simulink model "Z_1Dctrl"  (R2023a)
settings: Solver=ode1  StartTime=0.0  StopTime=inf  FixedStep=0.001  RelTol=1e-3  EnableMultiTasking=on
PostLoadFcn:
  | , if any(exist('dsrtsu_mdlpostloadfcn', 'file') ~= 0), dsrtsu_mdlpostloadfcn('Execute', bdroot); end,
InitFcn:
  | , if any(exist('rtifpga_mdlclblib', 'file') ~= 0), rtifpga_mdlclblib('Init', bdroot); end,
  | [b,a] = butter(6,0.6)
  | z0_default = 0.080001
  | fatness_default = 1
  | offset_default = 0
  | scale_default = 0
  | tic
model workspace (MAT data in the model file):
  Iters = 5
  N_coils = 6
  fatness_default = 1
  running = 0
  z0_default = 0.080001
undefined symbols (not defined in the file): a, b, DiscIntNeverNeededParam
libraries: dspstat3 x11, simulink x5, commfilt2 x4, rti2004lib x3, rtilibm x1
(part 2 of 2)

== system Z_1Dctrl/get_plant_input/detect_stability/speed_and_position_testing_xy ==
  x : Inport
  y : Inport  Port=2
  speed analysis : Subsystem
  |vxy| comfort threshold : Constant  Value=1e-6
  x_converged : Outport
  y_converged : Outport  Port=2
  wires:
  x/1 -> speed analysis/1(x)
  |vxy| comfort threshold/1 -> speed analysis/3(vxy comfort threshold)
  speed analysis/2(vy low enough) -> y_converged/1
  speed analysis/1(vx low enough) -> x_converged/1
  y/1 -> speed analysis/2(y)

== system Z_1Dctrl/plant/Position Determination1/XY position Calculation ==
  note: !!MODIFIED!!
      | Before: "X_p, Y_p = Head2_read, Head3_read - radius_m".
      | After: "Head2_p, Head3_p = Head2_read, Head3_read + radius_m".
  note: Laser sensors output a voltage in [-10,10]V, proportional to the detected object's position in their 40mm FOV.
      | Conventions:
      | - Top of sensor (with large chamfer) is "up". Bottom of sensor is "down".
      | - "Upmost" measurement is -10V (-0.02m).
      | - "Downmost" measurement is +10V (+0.02m).
      | - Measurements go wonky if outer boundaries (+10V, -10V) are reached. For safety, do not let the magnet reach this range.
  Head II (Voltage) : Inport
  Head III (Voltage) : Inport  Port=2
  diameter_m : Inport  Port=3
  Mux : Mux  Inputs=2
  Sum : Sum  Inputs=|++
  Sum1 : Sum  Inputs=++|
  X_m : Fcn  Expr=(u(1)+u(2))*sin(pi/4)
  Y_m : Fcn  Expr=(u(1)-u(2))*sin(pi/4)
  diameter_to_radius : Gain  Gain=1/2
  volt_to_m : Gain  Gain=2/1000
  volt_to_m_2 : Gain  Gain=2/1000
  X_Position(m) : Outport
  Y_Position(m) : Outport  Port=2
  wires:
  Head III (Voltage)/1 -> volt_to_m_2/1
  Y_m/1 -> Y_Position(m)/1
  X_m/1 -> X_Position(m)/1
  Head II (Voltage)/1 -> volt_to_m/1
  Mux/1 -> Y_m/1, X_m/1
  Sum1/1 -> Mux/2  "Head3_p"
  volt_to_m_2/1 -> Sum1/2
  Sum/1 -> Mux/1  "Head2_p"
  diameter_to_radius/1 -> Sum1/1, Sum/2  "radius_m"
  volt_to_m/1 -> Sum/1
  diameter_m/1 -> diameter_to_radius/1

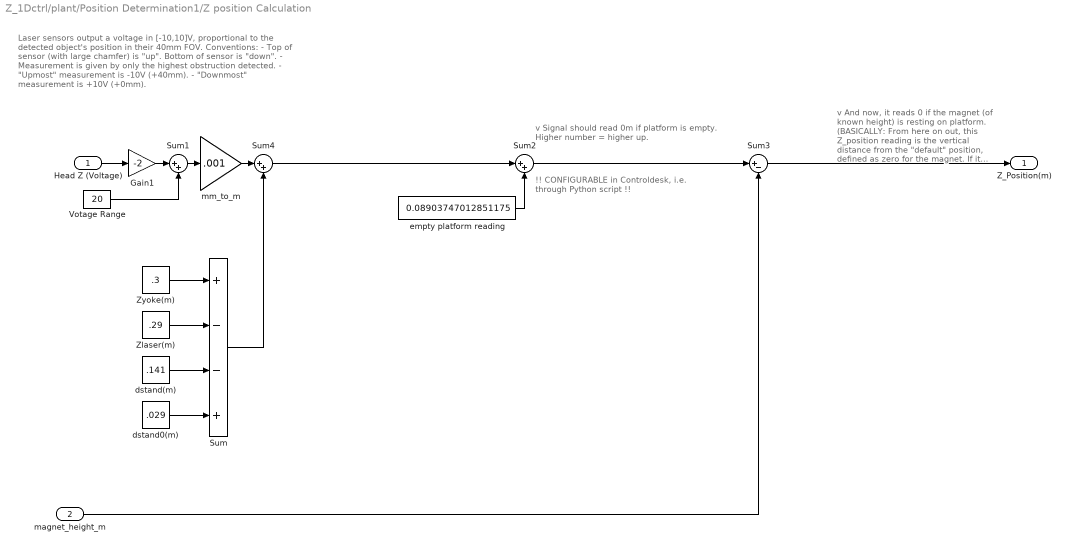
== system Z_1Dctrl/plant/Position Determination1/Z position Calculation ==
  note: Laser sensors output a voltage in [-10,10]V, proportional to the detected object's position in their 40mm FOV.
      | Conventions:
      | - Top of sensor (with large chamfer) is "up". Bottom of sensor is "down".
      | - Measurement is given by only the highest obstruction detected.
      | - "Upmost" measurement is -10V (+40mm).
      | - "Downmost" measurement is +10V (+0mm).
  note: v Signal should read 0m if platform is empty.
      | Higher number = higher up.
  note: v And now, it reads 0 if the magnet (of known height) is resting on platform.
      |
      | (BASICALLY: From here on out, this Z_position reading is the vertical distance from the "default" position, defined as zero for the magnet. If it reads something significantly different from 0, then double check the magnet height.)
  note: !! CONFIGURABLE in Controldesk, i.e. through Python script !!
  Head Z (Voltage) : Inport
  magnet_height_m : Inport  Port=2
  Gain1 : Gain  Gain=-2
  Sum : Sum  Inputs=+--+
  Sum1 : Sum  Inputs=|++
  Sum2 : Sum  Inputs=|++
  Sum3 : Sum  Inputs=|+-
  Sum4 : Sum  Inputs=|++
  Votage Range : Constant  Value=20
  Zlaser(m) : Constant  Value=.29
  Zyoke(m) : Constant  Value=.3
  dstand(m) : Constant  Value=.141
  dstand0(m) : Constant  Value=.029
  empty platform reading : Constant  Value=0.08903747012851175
  mm_to_m : Gain  Gain=.001
  Z_Position(m) : Outport
  wires:
  Sum2/1 -> Sum3/1
  Head Z (Voltage)/1 -> Gain1/1
  Sum/1 -> Sum4/2
  Sum1/1 -> mm_to_m/1
  Votage Range/1 -> Sum1/2
  Gain1/1 -> Sum1/1
  Zlaser(m)/1 -> Sum/2
  Zyoke(m)/1 -> Sum/1
  dstand(m)/1 -> Sum/3
  dstand0(m)/1 -> Sum/4
  magnet_height_m/1 -> Sum3/2
  Sum4/1 -> Sum2/1
  mm_to_m/1 -> Sum4/1
  empty platform reading/1 -> Sum2/2
  Sum3/1 -> Z_Position(m)/1

== system Z_1Dctrl/plant/Position Determination1/x filter ==
  u_raw : Inport
  10ms mean : Subsystem
  butter : DiscreteTransferFcn  Numerator=b  Denominator=a
  enable_butterworth : Constant
  enable_moving_mean : Constant
  switch_butter : Switch  Criteria=u2 > Threshold  SaturateOnIntegerOverflow=off  InputSameDT=off
  switch_movingmean : Switch  Criteria=u2 > Threshold  SaturateOnIntegerOverflow=off  InputSameDT=off
  u_filtered : Outport
  wires:
  enable_butterworth/1 -> switch_butter/2
  butter/1 -> switch_butter/1
  u_raw/1 -> switch_butter/3, butter/1
  enable_moving_mean/1 -> switch_movingmean/2
  switch_butter/1 -> 10ms mean/1(u), switch_movingmean/3
  10ms mean/1(movingmean(u)) -> switch_movingmean/1
  switch_movingmean/1 -> u_filtered/1

== system Z_1Dctrl/plant/Position Determination1/y filter ==
  u_raw : Inport
  10ms mean : Subsystem
  butter : DiscreteTransferFcn  Numerator=b  Denominator=a
  enable_butterworth : Constant
  enable_moving_mean : Constant
  switch_butter : Switch  Criteria=u2 > Threshold  SaturateOnIntegerOverflow=off  InputSameDT=off
  switch_movingmean : Switch  Criteria=u2 > Threshold  SaturateOnIntegerOverflow=off  InputSameDT=off
  u_filtered : Outport
  wires:
  enable_butterworth/1 -> switch_butter/2
  butter/1 -> switch_butter/1
  u_raw/1 -> switch_butter/3, butter/1
  enable_moving_mean/1 -> switch_movingmean/2
  switch_butter/1 -> 10ms mean/1(u), switch_movingmean/3
  10ms mean/1(movingmean(u)) -> switch_movingmean/1
  switch_movingmean/1 -> u_filtered/1

== system Z_1Dctrl/plant/Position Determination1/z filter RAW ==
  note: Leave filters OFF.
  u_raw : Inport
  u_filtered : Outport
  wires:
  u_raw/1 -> u_filtered/1

== system Z_1Dctrl/plant/Position Determination1/z filter SMOOTH ==
  u_raw : Inport
  10ms mean : Subsystem
  Terminator : Terminator  Commented=on
  Wn : Constant  Commented=on  Value=0.6
  butter : DiscreteTransferFcn  Numerator=b  Denominator=a
  butter2 : DiscreteTransferFcn  Commented=on  NumeratorSource=Input port  Numerator=b  DenominatorSource=Input port  Denominator=a  a0EqualsOne=on
      settings: InputPortMap=u0,p1,p3
  butterworth : MATLAB Function  Commented=on  TreatAsAtomicUnit=on
  enable_butterworth : Constant
  enable_moving_mean : Constant
  std_z : dspstat3/Moving Standard Deviation  Commented=on  Method=Sliding window  ForgettingFactorPort=off  SpecifyWindowLength=on  WindowLength=1000  OverlapLength=999  AllowArbitraryInputLength=off  ForgettingFactor=0.9  SimulateUsing=Code generation
  switch_butter : Switch  Criteria=u2 > Threshold  SaturateOnIntegerOverflow=off  InputSameDT=off
  switch_movingmean : Switch  Criteria=u2 > Threshold  SaturateOnIntegerOverflow=off  InputSameDT=off
  u_filtered : Outport
  wires:
  enable_butterworth/1 -> switch_butter/2
  u_raw/1 -> butter/1, switch_butter/3
  enable_moving_mean/1 -> switch_movingmean/2
  switch_butter/1 -> 10ms mean/1(u), switch_movingmean/3
  10ms mean/1(movingmean(u)) -> switch_movingmean/1
  switch_movingmean/1 -> std_z/1, u_filtered/1
  Wn/1 -> butterworth/1(Wn)
  butterworth/2(aye) -> butter2/3
  butterworth/1(bee) -> butter2/2
  butter2/1 -> ?
  std_z/1 -> Terminator/1
  butter/1 -> switch_butter/1

== system Z_1Dctrl/plant/output signal/output signal diagnostics ==
  H123_raw : Inport
  Discrete Transfer Fcn3 : DiscreteTransferFcn  NumeratorSource=Input port  Numerator=b  DenominatorSource=Input port  Denominator=a  a0EqualsOne=on
      settings: InputPortMap=u0,p1,p3
  Filtered signals : Demux  Outputs=3
  Mux : Mux  Inputs=3
  Raw signals : Demux  Outputs=3
  STDs : Subsystem
  Terminator1 : Terminator
  Terminator2 : Terminator
  Terminator3 : Terminator
  Wn : Constant  Value=0.9
  butterworth : MATLAB Function  TreatAsAtomicUnit=on
  center : Subsystem
  order : Constant  Value=6
  wires:
  Filtered signals/2 -> Terminator2/1  "HII_cen_fil"
  Filtered signals/3 -> Terminator3/1  "HIII_cen_fil"
  butterworth/1(bee) -> Discrete Transfer Fcn3/2
  butterworth/2(aye) -> Discrete Transfer Fcn3/3
  Discrete Transfer Fcn3/1 -> STDs/1(H123), Filtered signals/1
  order/1 -> butterworth/1(order)
  Wn/1 -> butterworth/2(Wn)
  H123_raw/1 -> center/1(u)
  Raw signals/1 -> Mux/1  "HZ_cen_raw"
  Raw signals/2 -> Mux/2  "HII_cen_raw"
  Raw signals/3 -> Mux/3  "HIII_cen_raw"
  Mux/1 -> Discrete Transfer Fcn3/1
  Filtered signals/1 -> Terminator1/1  "HZ_cen_fil"
  center/1(u_cen) -> Raw signals/1  "H123_cen_raw"

== system Z_1Dctrl/RTI Data/RTI Data Store/RTI Data Store/RTI Data Store ==
  RTI Data Store : Subsystem  mask(RTI_DATA_STORE){}
      mask help:
      | RTI Data Store Block. This block is used by RTI to store internal model dependent data. Deleting this block will result in data loss.
      |
      | NEVER DELETE, COPY, OR MODIFY THIS BLOCK!
      mask Help:
      | RTI Data Store Block. This block is used by RTI to store internal model dependent data. Deleting this block will result in data loss.
      | 
      | NEVER DELETE, COPY, OR MODIFY THIS BLOCK!
      mask Display: text(0.5, 0.5, ' ', 'HorizontalAlignment', 'center');

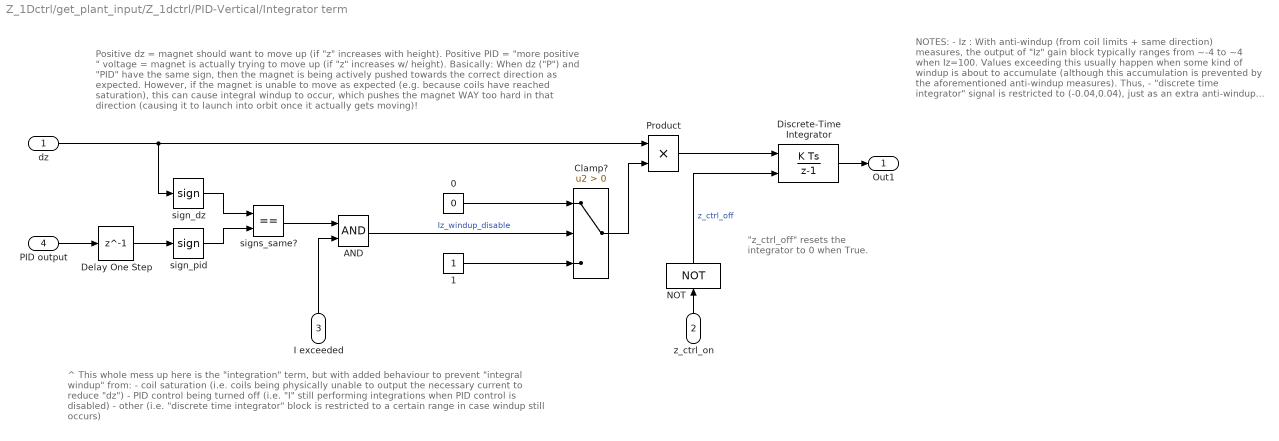
== system Z_1Dctrl/get_plant_input/Z_1dctrl/PID-Vertical/Integrator term ==
  note: "z_ctrl_off" resets the integrator to 0 when True.
  note: Positive dz = magnet should want to move up (if "z" increases with height).
      | Positive PID = "more positive " voltage = magnet is actually trying to move up (if "z" increases w/ height).
      |
      | Basically: When dz ("P") and "PID" have the same sign, then the magnet is being actively pushed towards the correct direction as expected. However, if the magnet is unable to move as expected (e.g. because coils have reached saturation), this can cause integral windup to occur, which pushes the magnet WAY too hard in that direction (causing it to launch into orbit once it actually gets moving)!
  note: NOTES:
      | - Iz : With anti-windup (from coil limits + same direction) measures, the output of "Iz" gain block typically ranges from ~-4 to ~4 when Iz=100. Values exceeding this usually happen when some kind of windup is about to accumulate (although this accumulation is prevented by the aforementioned anti-windup measures).
      | Thus,
      | - "discrete time integrator" signal is restricted to (-0.04,0.04), just as an extra anti-windup measure.
      | - Also, the integral resets while z-control is disabled.
  note: ^ This whole mess up here is the "integration" term, but with added behaviour to prevent "integral windup" from:
      | - coil saturation (i.e. coils being physically unable to output the necessary current to reduce "dz")
      | - PID control being turned off (i.e. "I" still performing integrations when PID control is disabled)
      | - other (i.e. "discrete time integrator" block is restricted to a certain range in case windup still occurs)
  dz : Inport
  z_ctrl_on : Inport  Port=2
  I exceeded : Inport  Port=3
  PID output : Inport  Port=4
  0 : Constant  Value=0
  1 : Constant
  AND : Logic  AllPortsSameDT=off  OutDataTypeStr=boolean
  Clamp? : Switch  Criteria=u2 > Threshold  SaturateOnIntegerOverflow=off  InputSameDT=off
  Delay One Step : Delay  DelayLength=1
  Discrete-Time Integrator : DiscreteIntegrator  ExternalReset=sampled level  SampleTime=-1  LimitOutput=on  UpperSaturationLimit=0.04  LowerSaturationLimit=-0.04  ICPrevOutput=DiscIntNeverNeededParam  ICPrevScaledInput=DiscIntNeverNeededParam
  NOT : Logic  Operator=NOT  AllPortsSameDT=off  OutDataTypeStr=boolean
  Product : Product
  sign_dz : Signum
  sign_pid : Signum
  signs_same? : RelationalOperator  Operator===  OutDataTypeStr=boolean  RndMeth=Simplest  InputSameDT=off
  Out1 : Outport
  wires:
  sign_dz/1 -> signs_same?/1
  AND/1 -> Clamp?/2  "Iz_windup_disable"
  signs_same?/1 -> AND/1
  sign_pid/1 -> signs_same?/2
  1/1 -> Clamp?/3
  NOT/1 -> Discrete-Time Integrator/2  "z_ctrl_off"
  0/1 -> Clamp?/1
  Product/1 -> Discrete-Time Integrator/1
  dz/1 -> sign_dz/1, Product/1
  Clamp?/1 -> Product/2
  PID output/1 -> Delay One Step/1
  Discrete-Time Integrator/1 -> Out1/1
  z_ctrl_on/1 -> NOT/1
  I exceeded/1 -> AND/2
  Delay One Step/1 -> sign_pid/1

== system Z_1Dctrl/get_plant_input/Z_1dctrl/PID-Vertical/PID Gain scheduler ==
  Zd : Inport
  dz : Inport  Port=2
  Dz : Constant  Value=nan
  Iz : Constant  Value=nan
  PID selector : MATLAB Function  TreatAsAtomicUnit=on
  Pz : Constant  Value=nan
  "[Pz, Iz, Dz_outer, Dz_inner, z] array" : Constant  Value=[400 2000 3200 3200 0.002; 310 350 5500 4000 0.005]
  dz_inner_threshold_mm : Constant  Value=0.1
  dz_outer_threshold_mm : Constant  Value=0.25
  PID_gains : Outport
  wires:
  Zd/1 -> PID selector/1(Zd)
  Iz/1 -> PID selector/7(I_override)
  Dz/1 -> PID selector/8(D_override)
  dz/1 -> PID selector/2(dz)
  dz_outer_threshold_mm/1 -> PID selector/5(dz_outer_threshold)
  "[Pz, Iz, Dz_outer, Dz_inner, z] array"/1 -> PID selector/3(PIDDz_save)
  Pz/1 -> PID selector/6(P_override)
  dz_inner_threshold_mm/1 -> PID selector/4(dz_inner_threshold)
  PID selector/1(PID_out) -> PID_gains/1

== system Z_1Dctrl/get_plant_input/detect_stability/speed_and_position_testing/convergence analysis ==
  dz : Inport
  dz convergence threshold : Inport  Port=2
  dz comfort threshold : Inport  Port=3
  GreaterThanOrEqual1 : RelationalOperator  Operator=<=  OutDataTypeStr=boolean  RndMeth=Simplest  InputSameDT=off
  GreaterThanOrEqual2 : RelationalOperator  Operator=<=  OutDataTypeStr=boolean  RndMeth=Simplest  InputSameDT=off
  Maximum |dz| over 100ms : dspstat3/Moving Maximum  SpecifyWindowLength=on  WindowLength=100  SimulateUsing=Code generation
  z_equals_Zd : Outport
  z_closeto_Zd : Outport  Port=2
  wires:
  GreaterThanOrEqual1/1 -> z_equals_Zd/1  "z_converged"
  dz/1 -> Maximum |dz| over 100ms/1
  dz convergence threshold/1 -> GreaterThanOrEqual1/2
  Maximum |dz| over 100ms/1 -> GreaterThanOrEqual1/1, GreaterThanOrEqual2/1
  GreaterThanOrEqual2/1 -> z_closeto_Zd/1  "z_closeenough"
  dz comfort threshold/1 -> GreaterThanOrEqual2/2

== system Z_1Dctrl/get_plant_input/detect_stability/speed_and_position_testing/position analysis ==
  dz : Inport
  dz comfort threshold : Inport  Port=2
  GreaterThanOrEqual2 : RelationalOperator  Operator=<=  OutDataTypeStr=boolean  RndMeth=Simplest  InputSameDT=off
  z_closeenough : Outport
  wires:
  dz/1 -> GreaterThanOrEqual2/1
  GreaterThanOrEqual2/1 -> z_closeenough/1  "z_closeenough"
  dz comfort threshold/1 -> GreaterThanOrEqual2/2

== system Z_1Dctrl/get_plant_input/detect_stability/speed_and_position_testing/speed analysis ==
  note: NOTE:
      | When Zd changes gradually, the speed peaks tend to go up from ~2e-6m/ms to around ~1e-5 m/ms.
      | When Zd changes suddenly, the speed peaks tend to jump up to ~2e-5m/ms per millimetre difference in Zd (e.g. going from Zd=2mm to Zd=3mm would record a speed peak of around ~4e-5m/ms).
      |
      | When the magnet has a set Zd and coil perturbations gradually change, the speed peaks are basically unchanged.
      | When the magnet has a set Zd and coil perturbations suddenly change, speed peaks can exceed ~1e-5m/ms very easily.
      |
      | Thus: 5e-6 m/ms seems to be a good line beyond which speed peaks indicate either intentional vertical movement OR an unwanted z-jitter during horizontal movement. When this occurs will be tracked using a moving maximum over some short timeframe (~100ms?).
      |
      | ** The above is WITH "z" being the 10ms average of the raw signal. Changing this may require recalibration of this speed threshold. **
  z : Inport
  vz comfort threshold : Inport  Port=2
  vz DANGER threshold : Inport  Port=3
  dz close enough : Inport  Port=4
  AND : Logic  AllPortsSameDT=off  OutDataTypeStr=boolean
  Maximum |vz| over 100ms : dspstat3/Moving Maximum  SpecifyWindowLength=on  WindowLength=100  SimulateUsing=Code generation
  NOT : Logic  Operator=NOT  IconShape=distinctive  AllPortsSameDT=off  OutDataTypeStr=boolean
  vz dangerously high : RelationalOperator  OutDataTypeStr=boolean  RndMeth=Simplest  InputSameDT=off
  vz uncomfortably high : RelationalOperator  OutDataTypeStr=boolean  RndMeth=Simplest  InputSameDT=off
  z - z_previous : simulink/Discrete/Difference  ICPrevInput=0.0  OutMin=[]  OutMax=[]  OutDataType=fixdt(1, 16)  OutScaling=2^-10  DoSatur=off
  |z - z_previous| : Abs  SaturateOnIntegerOverflow=off
  vz jump detected : Outport
  vz DANGEROUSLY high : Outport  Port=2
  wires:
  z - z_previous/1 -> |z - z_previous|/1
  z/1 -> z - z_previous/1
  |z - z_previous|/1 -> Maximum |vz| over 100ms/1  "|z - z_prev|/dt (m/ms)"
  vz uncomfortably high/1 -> AND/1
  vz comfort threshold/1 -> vz uncomfortably high/2
  vz dangerously high/1 -> vz DANGEROUSLY high/1
  vz DANGER threshold/1 -> vz dangerously high/2
  dz close enough/1 -> NOT/1
  NOT/1 -> AND/2  "dz uncomfortably far?"
  AND/1 -> vz jump detected/1
  Maximum |vz| over 100ms/1 -> vz dangerously high/1, vz uncomfortably high/1

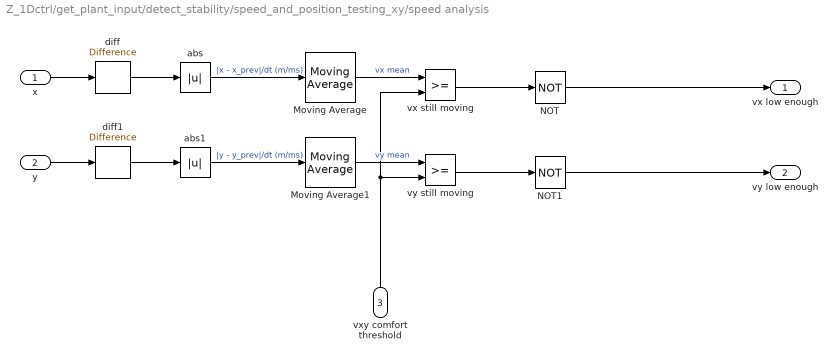
== system Z_1Dctrl/get_plant_input/detect_stability/speed_and_position_testing_xy/speed analysis ==
  x : Inport
  y : Inport  Port=2
  vxy comfort threshold : Inport  Port=3
  Moving Average : dspstat3/Moving Average  Method=Sliding window  ForgettingFactorPort=off  SpecifyWindowLength=on  WindowLength=100  OverlapLength=99  AllowArbitraryInputLength=off  ForgettingFactor=0.9  SimulateUsing=Code generation
  Moving Average1 : dspstat3/Moving Average  Method=Sliding window  ForgettingFactorPort=off  SpecifyWindowLength=on  WindowLength=100  OverlapLength=99  AllowArbitraryInputLength=off  ForgettingFactor=0.9  SimulateUsing=Code generation
  NOT : Logic  Operator=NOT  IconShape=distinctive  AllPortsSameDT=off  OutDataTypeStr=boolean
  NOT1 : Logic  Operator=NOT  IconShape=distinctive  AllPortsSameDT=off  OutDataTypeStr=boolean
  abs : Abs  SaturateOnIntegerOverflow=off
  abs1 : Abs  SaturateOnIntegerOverflow=off
  diff : simulink/Discrete/Difference  ICPrevInput=0.0  OutMin=[]  OutMax=[]  OutDataType=fixdt(1, 16)  OutScaling=2^-10  DoSatur=off
  diff1 : simulink/Discrete/Difference  ICPrevInput=0.0  OutMin=[]  OutMax=[]  OutDataType=fixdt(1, 16)  OutScaling=2^-10  DoSatur=off
  vx still moving : RelationalOperator  OutDataTypeStr=boolean  RndMeth=Simplest  InputSameDT=off
  vy still moving : RelationalOperator  OutDataTypeStr=boolean  RndMeth=Simplest  InputSameDT=off
  vx low enough : Outport
  vy low enough : Outport  Port=2
  wires:
  diff/1 -> abs/1
  x/1 -> diff/1
  abs/1 -> Moving Average/1  "|x - x_prev|/dt (m/ms)"
  vxy comfort threshold/1 -> vy still moving/2, vx still moving/2
  vy still moving/1 -> NOT1/1
  y/1 -> diff1/1
  vx still moving/1 -> NOT/1
  abs1/1 -> Moving Average1/1  "|y - y_prev|/dt (m/ms)"
  diff1/1 -> abs1/1
  NOT/1 -> vx low enough/1
  NOT1/1 -> vy low enough/1
  Moving Average/1 -> vx still moving/1  "vx mean"
  Moving Average1/1 -> vy still moving/1  "vy mean"

== system Z_1Dctrl/plant/Position Determination1/x filter/10ms mean ==
  note: NOTE: Sensor readings fluctuate over a peak-to-peak amplitude of about 4.5e-5 m, over a period of almost exactly 10ms.
      |
      | 08/14/23: See how it improves if I only consider the mean signal over 10ms!
  u : Inport
  ave signal : Product  Inputs=*/
  integration window (samples) : Constant  Value=10
  sum of signal over short time : commfilt2/Windowed Integrator  integperiod=10  InputProcessing=Columns as channels (frame based)  roundingMode=Floor  overflowMode=off  coeffDataTypeStr=Inherit: Same word length as input  coeffMin=[]  coeffMax=[]  coeffLastDataTypeStr=Inherit: Same word length as input  accumDataTypeStr=Inherit: Same as product output  accumLastDataTypeStr=Inherit: Same as product output  outputDataTypeStr=Inherit: Same as accumulator  outputMin=[]  outputMax=[]  outputLastDataTypeStr=Inherit: Same as accumulator
  movingmean(u) : Outport
  wires:
  sum of signal over short time/1 -> ave signal/1
  u/1 -> sum of signal over short time/1
  integration window (samples)/1 -> ave signal/2
  ave signal/1 -> movingmean(u)/1

== system Z_1Dctrl/plant/Position Determination1/y filter/10ms mean ==
  note: NOTE: Sensor readings fluctuate over a peak-to-peak amplitude of about 4.5e-5 m, over a period of almost exactly 10ms.
      |
      | 08/14/23: See how it improves if I only consider the mean signal over 10ms!
  u : Inport
  ave signal : Product  Inputs=*/
  integration window (samples) : Constant  Value=10
  sum of signal over short time : commfilt2/Windowed Integrator  integperiod=10  InputProcessing=Columns as channels (frame based)  roundingMode=Floor  overflowMode=off  coeffDataTypeStr=Inherit: Same word length as input  coeffMin=[]  coeffMax=[]  coeffLastDataTypeStr=Inherit: Same word length as input  accumDataTypeStr=Inherit: Same as product output  accumLastDataTypeStr=Inherit: Same as product output  outputDataTypeStr=Inherit: Same as accumulator  outputMin=[]  outputMax=[]  outputLastDataTypeStr=Inherit: Same as accumulator
  movingmean(u) : Outport
  wires:
  sum of signal over short time/1 -> ave signal/1
  u/1 -> sum of signal over short time/1
  integration window (samples)/1 -> ave signal/2
  ave signal/1 -> movingmean(u)/1

== system Z_1Dctrl/plant/Position Determination1/z filter SMOOTH/10ms mean ==
  note: NOTE: Sensor readings fluctuate over a peak-to-peak amplitude of about 4.5e-5 m, over a period of almost exactly 10ms.
      |
      | 08/14/23: See how it improves if I only consider the mean signal over 10ms!
  u : Inport
  ave signal : Product  Inputs=*/
  integration window (samples) : Constant  Value=10
  sum of signal over short time : commfilt2/Windowed Integrator  integperiod=10  InputProcessing=Columns as channels (frame based)  roundingMode=Floor  overflowMode=off  coeffDataTypeStr=Inherit: Same word length as input  coeffMin=[]  coeffMax=[]  coeffLastDataTypeStr=Inherit: Same word length as input  accumDataTypeStr=Inherit: Same as product output  accumLastDataTypeStr=Inherit: Same as product output  outputDataTypeStr=Inherit: Same as accumulator  outputMin=[]  outputMax=[]  outputLastDataTypeStr=Inherit: Same as accumulator
  movingmean(u) : Outport
  wires:
  sum of signal over short time/1 -> ave signal/1
  u/1 -> sum of signal over short time/1
  integration window (samples)/1 -> ave signal/2
  ave signal/1 -> movingmean(u)/1

== system Z_1Dctrl/plant/output signal/output signal diagnostics/STDs ==
  H123 : Inport
  Demux : Demux  Outputs=3
  Moving Standard Deviation : dspstat3/Moving Standard Deviation  Method=Sliding window  ForgettingFactorPort=off  SpecifyWindowLength=on  WindowLength=3000  OverlapLength=2999  AllowArbitraryInputLength=off  ForgettingFactor=0.9  SimulateUsing=Code generation
  Moving Standard Deviation1 : dspstat3/Moving Standard Deviation  Method=Sliding window  ForgettingFactorPort=off  SpecifyWindowLength=on  WindowLength=3000  OverlapLength=2999  AllowArbitraryInputLength=off  ForgettingFactor=0.9  SimulateUsing=Code generation
  Moving Standard Deviation2 : dspstat3/Moving Standard Deviation  Method=Sliding window  ForgettingFactorPort=off  SpecifyWindowLength=on  WindowLength=3000  OverlapLength=2999  AllowArbitraryInputLength=off  ForgettingFactor=0.9  SimulateUsing=Code generation
  Terminator : Terminator
  Terminator1 : Terminator
  Terminator2 : Terminator
  wires:
  H123/1 -> Demux/1
  Demux/1 -> Moving Standard Deviation/1
  Demux/2 -> Moving Standard Deviation1/1
  Demux/3 -> Moving Standard Deviation2/1
  Moving Standard Deviation/1 -> Terminator/1  "std_HZ"
  Moving Standard Deviation1/1 -> Terminator1/1  "std_HII"
  Moving Standard Deviation2/1 -> Terminator2/1  "std_HIII"

== system Z_1Dctrl/plant/output signal/output signal diagnostics/center ==
  u : Inport
  Demux : Demux  Outputs=3
  Moving Average : dspstat3/Moving Average  Method=Sliding window  ForgettingFactorPort=off  SpecifyWindowLength=on  WindowLength=1000  OverlapLength=999  AllowArbitraryInputLength=off  ForgettingFactor=0.9  SimulateUsing=Code generation
  Moving Average1 : dspstat3/Moving Average  Method=Sliding window  ForgettingFactorPort=off  SpecifyWindowLength=on  WindowLength=1000  OverlapLength=999  AllowArbitraryInputLength=off  ForgettingFactor=0.9  SimulateUsing=Code generation
  Moving Average2 : dspstat3/Moving Average  Method=Sliding window  ForgettingFactorPort=off  SpecifyWindowLength=on  WindowLength=1000  OverlapLength=999  AllowArbitraryInputLength=off  ForgettingFactor=0.9  SimulateUsing=Code generation
  Mux : Mux  Inputs=3
  Sum : Sum  Inputs=|+-
  Sum1 : Sum  Inputs=|+-
  Sum2 : Sum  Inputs=|+-
  u_cen : Outport
  wires:
  u/1 -> Demux/1
  Moving Average/1 -> Sum/2
  Demux/1 -> Sum/1, Moving Average/1
  Moving Average1/1 -> Sum1/2
  Demux/2 -> Moving Average1/1, Sum1/1
  Moving Average2/1 -> Sum2/2
  Demux/3 -> Moving Average2/1, Sum2/1
  Sum1/1 -> Mux/2
  Sum/1 -> Mux/1
  Sum2/1 -> Mux/3
  Mux/1 -> u_cen/1

== system Z_1Dctrl/RTI Data/RTI Data Store/RTI Data Store/RTI Data Store/RTI Data Store ==

== matlab function Z_1Dctrl/get_plant_input/Z_1dctrl/PID-Vertical/PID Gain scheduler/PID selector ==
  data: Zd input; dz input; PIDDz_save input; dz_inner_threshold input; dz_outer_threshold input; PID_out output; P_override input; I_override input; D_override input
function PID_out = fcn(Zd,dz,PIDDz_save,dz_inner_threshold, dz_outer_threshold, P_override,I_override,D_override)
% Interpolates for PID gains based on target Zd, using PID gains that were
% manually tuned at various target heights (with D gain being split into
% "near target height" and "far from target height" values, to allow for
% strong D contribution without risking destabilization near convergence).
% The "D" gain is then chosen between these aforementioned values based on
% how near/far the magnet is to Zd.
%
% Finally, overri

% Read recorded PID gains
Zq = Zd;

Ps = PIDDz_save(:,1);
Is = PIDDz_save(:,2);
Douts = PIDDz_save(:,3);
Dins = PIDDz_save(:,4);
Zs = PIDDz_save(:,5);
[~,lowest_index] = min(Zs);
[~,highest_index] = max(Zs);


% Interpolate if necessary!
if Zd <= Zs(lowest_index)
    % disp("Below 2mm!")
    P_final = Ps(lowest_index);
    I_final = Is(lowest_index);
    Dout_final = Douts(lowest_index);
    Din_final  = Dins(lowest_index);
elseif Zd >= Zs(highest_index)
    % disp("Above 5mm!")
    P_final = Ps(highest_index);
    I_final = Is(highest_index);
    Dout_final = Douts(highest_index);
    Din_final  = Dins(highest_index);
else
    % disp("Interpolate!")
    P_final     = interp1(Zs,Ps,Zq,'spline');
    I_final     = interp1(Zs,Is,Zq,'spline');
    Dout_final  = interp1(Zs,Douts,Zq,'spline');
    Din_final   = interp1(Zs,Dins,Zq,'spline');
end



% Choose between "inner" and "outer" D gains
dz_mm = dz * 1000;

if abs(dz_mm) <= dz_inner_threshold
    % disp("Within inner threshold")
    D_final = Din_final;
elseif abs(dz_mm) >= dz_outer_threshold
    % disp("Beyond outer threshold")
    D_final = Dout_final;
else
    % disp("In between; interpolate!")
    D_final = ( Dout_final- Din_final)*(abs(dz_mm) - dz_inner_threshold)/(dz_outer_threshold - dz_inner_threshold) +  Din_final;
end


% Apply overrides (if any)
if ~isnan(P_override)
    P_final = P_override;
end
if ~isnan(I_override)
    I_final = I_override;
end
if ~isnan(D_override)
    D_final = D_override;
end
PID_out = [P_final, I_final, D_final];

== matlab function Z_1Dctrl/plant/output signal/output signal diagnostics/butterworth ==
  data: order input; bee output; Wn input; aye output
function [bee,aye] = butterwort(order,Wn)
% order = order of lowpass Butterworth filter
% Wn = NORMALIZED cutoff frequency
%    = fc/(fs/2), where fc = cutoff frequency (Hz),
%                       fs = sample frequency (Hz) (1000 for our system)
%    = ratio between cutoff frequency and HALF of sample frequency!

% Ignore the order actually lmao
order = 2;
[bee,aye] = butter(order,Wn);

== matlab function Z_1Dctrl/plant/Position Determination1/z filter SMOOTH/butterworth ==
  data: bee output; Wn input; aye output
function [bee,aye] = butterwort(Wn)
% order = order of lowpass Butterworth filter
% Wn = NORMALIZED cutoff frequency
%    = fc/(fs/2), where fc = cutoff frequency (Hz),
%                       fs = sample frequency (Hz) (1000 for our system)
%    = ratio between cutoff frequency and HALF of sample frequency!

% Ignore the order actually lmao
order = 6;
[bee,aye] = butter(order,Wn);

== matlab function Z_1Dctrl/Input parameters/Magnet Specs/Magnet Physical Specs ==
  data: unit_mode input; diameter input; height input; diameter_m output; height_m output; mass_g output; B_r output; mass input; magnet_remanence_t input; errorflag output
function [diameter_m,height_m,mass_g,B_r,errorflag]= mag_specs(unit_mode,diameter,height,mass,magnet_remanence_t)
% User can specify parameters for cylindrical magnets: diameter, height 
% (units: "in" or "cm" or "mm" or "m"), mass, and either remanent B-field
% (in T or G) or magnetic dipole moment (in N*m/T, aka A*m^2).
% TO IMPLEMENT: Ring magnets!

errorflag = 0;

%%% DIMENSIONS %%%
% Dimensions, in m
% NOTE: Unit modes are:
% 1 - m
% 2 - cm
% 3 - mm
% 4 - in
if unit_mode==1
    units_to_m = 1;
elseif unit_mode==2
    units_to_m = 0.01;
elseif unit_mode==3
    units_to_m = 0.001;
elseif unit_mode==4
    units_to_m = 0.0254;
else
    % (TEMP?) Assume that the user wants metres
    units_to_m = 1;
end

% Dimensions
% if isnan(diameter)
%     diameter = diameter_detect;
% end
% if isnan(diameter_detect)
%     diameter_detect = diameter;
% end
% if isnan(height)
%     height = height_detect;
% end
% if isnan(height_detect)
%     height_detect = height;
% end
diameter_m = diameter * units_to_m;
height_m = height * units_to_m;
mass_g = mass;

%%% MAG FIELD STUFF %%%
% Mag field info (Br in Gauss or T)
if magnet_remanence_t > 1000
    % Assumes a remanence field value based on the material, in Gauss.
    % For example, an N52 magnet has 14800G, and Xiaodong's now-battered
    % magnet has 12900G.
    B_r = magnet_remanence_t / 10000;
else
    % Assumes a remanence field value based on the material, in T.
    % For example, an N52 magnet has 1.48T, and Xiaodong's now-battered
    % magnet has 1.29T.
    B_r = magnet_remanence_t / 1;
end

% (!!!!) CREATE CHART FOR CONVERSION FROM Nxx FORMAT TO REMANENCE IN T

% K&J SPECS:
%     % Assumes a grade was inputted as a string-- N52, N42, etc!
%     if lower(magfield_grade_t)=="n52"
%         B_r = 1.48;
%     elseif lower(magfield_grade_t)=="n50"
%         B_r = 1.45;
%     elseif lower(magfield_grade_t)=="n48"
%         B_r = 1.42;
%     elseif lower(magfield_grade_t)=="n45"
%         B_r = 1.35;
%     elseif lower(magfield_grade_t)=="n42"
%         B_r = 1.32;
%     elseif lower(magfield_grade_t)=="n40"
%         B_r = 1.29;
%     elseif lower(magfield_grade_t)=="n35"
%         B_r = 1.21;
%     else
%         % SHOULD NEVER HAPPEN
%         B_r = 1.48;
%         errorflag = 1;
%     end
% APPLIEDMAGNETS SPECS:
%     % Assumes a grade was inputted as a string-- N52, N42, etc!
%     if lower(magfield_grade_t)=="n52"
%         B_r = 1.48;
%     elseif lower(magfield_grade_t)=="n50"
%         B_r = 1.45;
%     elseif lower(magfield_grade_t)=="n48"
%         B_r = 1.42;
%     elseif lower(magfield_grade_t)=="n45"
%         B_r = 1.38 (rarely 1.35);
%     elseif lower(magfield_grade_t)=="n42"
%         B_r = 1.32;
%     elseif lower(magfield_grade_t)=="n40"
%         B_r = 1.29;
%     else
%         % SHOULD NEVER HAPPEN
%         B_r = 1.48;
%         errorflag = 1;
%     end
% 
% 
%

== matlab function Z_1Dctrl/Monitoring/diagnostics ==
  data: magnet_specs output; magnet_specs input; xyz input; signal_raw input; xy_dangerzone_radiusfraction input; h123_off_minmax input; h123_empty_minmax input; z_rest_minmax input; h1_off output; h2_off output; h3_off output; h1_empty output; h2_or_h3_empty output; z_resting output; z_resting_too_low output; in_workspace output; xy_dangerzone output
function [magnet_specs, h1_off, h2_off, h3_off, h1_empty, h2_or_h3_empty, z_resting, z_resting_too_low, in_workspace, xy_dangerzone] = get_status(magnet_specs, xyz, signal_raw, xy_dangerzone_radiusfraction, ...
    h123_off_minmax, h123_empty_minmax, z_rest_minmax)
% Detects state of the magnet and/or laser sensors based on position data.
% Assumes that the values thresholds (i.e. inputs, such as h123_off_minmax)
% have already been calibrated beforehand.
%
% The resulting ``status" can then be read by ControlDesk and/or Python.
    height_m = magnet_specs(2);
    diameter_m = magnet_specs(1);
    x = xyz(1);
    y = xyz(2);
    z = xyz(3);
    head1_raw = signal_raw(1);
    head2_raw = signal_raw(2); % (sic)
    head3_raw = signal_raw(3); % (sic)

    h1_off_min = min(h123_off_minmax(1:2));
    h1_off_max = max(h123_off_minmax(1:2));
    h2_off_min = min(h123_off_minmax(3:4));
    h2_off_max = max(h123_off_minmax(3:4));
    h3_off_min = min(h123_off_minmax(5:6));
    h3_off_max = max(h123_off_minmax(5:6));

    h1_empty_min = min(h123_empty_minmax(1:2));
    h1_empty_max = max(h123_empty_minmax(1:2));
    h2_empty_min = min(h123_empty_minmax(3:4));
    h2_empty_max = max(h123_empty_minmax(3:4));
    h3_empty_min = min(h123_empty_minmax(5:6));
    h3_empty_max = max(h123_empty_minmax(4:6));

    % Detect on/off/empty/etc for each reading
    h1_off = head1_raw > h1_off_min && head1_raw < h1_off_max;
    h2_off = head2_raw > h2_off_min && head2_raw < h2_off_max;
    h3_off = head3_raw > h3_off_min && head3_raw < h3_off_max;

    h1_empty = head1_raw > h1_empty_min && head1_raw < h1_empty_max;
    h2_empty = head2_raw > h2_empty_min && head2_raw < h2_empty_max;
    h3_empty = head3_raw > h3_empty_min && head3_raw < h3_empty_max;
    h2_or_h3_empty = h2_empty || h3_empty;
    
    % Detect resting / levitating / etc
    z_rest_min = min(z_rest_minmax);
    z_rest_max = max(z_rest_minmax);
    z_resting = z > z_rest_min && z < z_rest_max;
    z_resting_too_low = z <= z_rest_min && z < z_rest_max ...
                  && z > -height_m && ~h1_empty;
    in_workspace =   ~(h1_off   && h2_off   && h3_off) ...
                  && (~h1_empty || ~h2_empty || ~h3_empty); % Edited 4/11/24
    % in_workspace =   ~(h1_off   && h2_off   && h3_off) ...
    %               && (~h1_empty || ~h2_empty || ~h3_empty) ...
    %               && (z > -height_m);

    % Detect whether XY is dangerously far from centre (i.e. Z-position
    % detection will soon be lost).
    radius_m = diameter_m / 2;

    % SELECT ONE OF THE FOLLOWING:
        % % Safe within fixed radius (not recommended; lots of wasted space):
        % xy_dangerzone_bool = norm([x,y]) > radius_m*xy_dangerzone_radiusfraction;

        % Safe within lasers' range (larger workspace, but slower training):
        xy_dangerzone_bool = (norm(x) > radius_m*xy_dangerzone_radiusfraction) || ...
                             (abs(head2_raw) < 1.00*xy_dangerzone_radiusfraction) || ...
                             (abs(head3_raw) < 1.00*xy_dangerzone_radiusfraction);
    xy_dangerzone = double(xy_dangerzone_bool);

== matlab function Z_1Dctrl/Monitoring/diagnostics_summary ==
  data: h1_off input; h2_off input; h3_off input; h1_empty input; h2_or_h3_empty input; z_resting input; z_resting_too_low input; in_workspace input; xy_dangerzone input; z_stable input; z_converged input; z_close input; vz_DANGER input; x_converged input; y_converged input; coils_saturated input; fully_off output; resting output; empty_workspace output; recording_safe output; e_stop input; quickreport output
function [fully_off, resting, empty_workspace, recording_safe, quickreport] = summarize_status(h1_off, h2_off, h3_off, h1_empty, h2_or_h3_empty, ...
    z_resting, z_resting_too_low, in_workspace, xy_dangerzone, z_stable, z_converged, z_close, vz_DANGER, x_converged, y_converged, coils_saturated, e_stop)
% Condenses diagnostic information. 
% The `diagnostic_quickreport` condenses all of this information into one
% integer via one-hot encoding.
%   000000000001 : ????
%   000000000010 : ????
%   000000000100 : Are coils saturated?
%   000000001000 : Is magnet's Y converged?
%   000000010000 : Is magnet's X converged?
%   000000100000 : Magnet resting status? (0, 1, 2, or 3; see "Detect resting...")
%   000001000000 : Is magnet's XY dangerously close to edge?
%   000010000000 : Is magnet converged?
%   000100000000 : Is magnet reasonably close to Zd?
%   001000000000 : Magnet stability status? (0=safe, 1=uncomfortable, 2=DANGER)
%   010000000000 : Is magnet detected by ALL sensors?
%   100000000000 : Is magnet detected by ANY sensor?
% 
% Notes for relevant info:
%     - are sensors off?
%     - is magnet resting?
%         - is magnet resting below XY sensors?
%     - is workspace empty?
%     - is there reason to stop RECORDING? e.g.:
%         - X readings empty
%         - Y readings empty
%         - Z readings empty
%         - Z not converged
%         - magnet resting on platform
%         - sensors off
%         - E-stop on

    % Detect off
    % 0 - sensors on
    % 1 - sensors off
    if h1_off && h2_off && h3_off
        fully_off = 1;
    else
        fully_off = 0;
    end

    % Detect resting on the platform
    % 0 - not on platform
    % 1 - on platform
    % 2 - on platform (XY not detected)
    % 3 - on platform ((!) NONSENSICALLY LOW)
    if z_resting_too_low
        resting = 3;
    elseif z_resting && (h2_or_h3_empty)
        resting = 2;
    elseif z_resting
        resting = 1;
    else
        resting = 0;
    end

    % Report z-stability status
    % (0=stable, 1=uncomfortable, 2=DANGER)
    if z_stable
        stability_status = 0;
    else
        stability_status = 1;
    end
    if vz_DANGER
        stability_status = 2;
    end

    % Detect empty workspace
    % 0 - not completely empty
    % 1 - completely empty
    empty_workspace = ~in_workspace;

    % Check if all sensors detect magnet
    is_ready_to_run = (~h1_empty && ~h2_or_h3_empty);   % Detected by ALL sensors

    % Check for reasons to stop recording
    if ~is_ready_to_run ...
            || fully_off || z_resting || z_resting_too_low ...
            || e_stop
        recording_safe = 0;
    else
        recording_safe = 1;
    end

    % Summary of all major statuses
    quickreport = ...
        100000000000 * in_workspace + ...
        010000000000 * (~h1_empty && ~h2_or_h3_empty) + ...
        001000000000 * stability_status + ...
        000100000000 * z_close + ...
        000010000000 * z_converged + ...
        000001000000 * xy_dangerzone + ...
        000000100000 * resting + ...
        000000010000 * x_converged + ...
        000000001000 * y_converged + ...
        000000000100 * coils_saturated;
    
        
end

== matlab function Z_1Dctrl/get_plant_input/Z_1dctrl/PID-Vertical/max(0,|dz|-threshold) ==
  data: u_threshold_mm input; u_m input; y output
function y = dz_past_threshold(u_threshold_mm, u_m)
% Input "u" is in metres.
% Input "u_threshold" is in mm.
u_mm = u_m * 1000;    
y = max(0,abs(u_mm) - u_threshold_mm);
